simulink model "testSerial"  (R2020a)
settings: Solver=ode3  StartTime=0.0  StopTime=inf  FixedStep=0.4  RelTol=1e-3
undefined symbols (not defined in the file or in its folder): CR, serial
libraries: instrumentlib x2
settings Model: Creator=vince  LastModifiedBy=vince

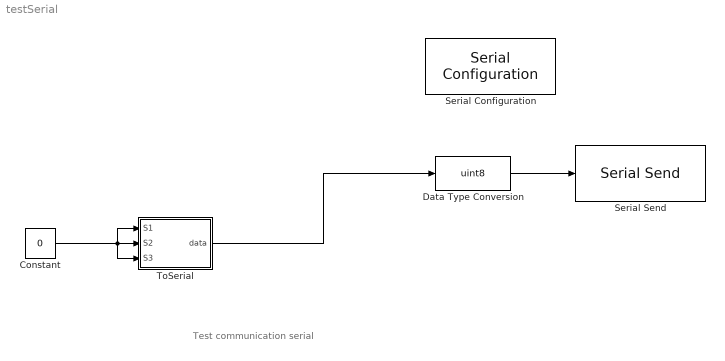
== system testSerial ==
  note: Test communication serial
  Constant : Constant  Value=0
  Data Type Conversion : DataTypeConversion  OutDataTypeStr=uint8
  Serial Configuration : instrumentlib/Serial Configuration  Priority=-200000  ComPortMenu=COM7  ComPort=COM7  ObjConstructor=serial('COM7');  BaudRate=9600  DataBits=8  Parity=none  StopBits=1  FlowControl=none  Timeout=10  ByteOrder=LittleEndian
  Serial Send : instrumentlib/Serial Send  ComPortMenu=COM7  ComPort=COM7  ObjConstructor=serial('COM7');  Terminator=CR ('\r')  EnableBlockingMode=off
  ToSerial : MATLAB Function  TreatAsAtomicUnit=on
  wires:
  Constant/1 -> ToSerial/1(S1), ToSerial/3(S3), ToSerial/2(S2)
  Data Type Conversion/1 -> Serial Send/1
  ToSerial/1(data) -> Data Type Conversion/1

== matlab function testSerial/ToSerial ==
  data: S1 input; data output double size=[1 3]; S2 input; S3 input
function data = ToSerial(S1,S2,S3)
data=zeros(1,3);
data(1)=S1(1);
data(2)=S2(1);
data(3)=S3(1);
